simulink model "kaiguangai1108"  (R2016b)
settings: Solver=ode4  StartTime=0.0  StopTime=inf  FixedStep=0.002  RelTol=1e-3  EnableMultiTasking=on
libraries: slrtlib x5
(part 3 of 6)

== stateflow chart kaiguangai1108/Subsystem1/zidong/1# ==
  state zidong
    state chushihua
      entry:
      skhx=0;
      kghx=0;
      kgzhiling1=0;
      kgzhiling2=0;
      yjhx=0;
      gghx=0;
      ggzhiling1=0;
      ggzhiling2=0;
      skt=0;
      kgt=0;
      sdt=0;
      jst=0;
      ggt=0;
      yjt=0;
      skyichang=0;
      kgyichang=0;
      sdyichang=0;
      jsyichang=0;
      ggyichang=0;
      yjyichang=0;
    state on1
      entry:
      skhx=1;
    state songkaishijian
      entry:
      skt=skt+0.002;
    state start
      entry:
      yikaicishu = 0;
    state on10
      entry:
      skyichang=1;
    state songkaishijian1
      entry:
      skt=skt+0.002;
    state on8
      entry:
      skhx=0;
    state yanchishijian1
      entry:
      t=t+0.002;
    state tguiling
      entry: t=0;
    state on2
      entry:
      skhx=0;
      kghx=1;
      kgzhiling1=1;
      kgzhiling2=1;
    state kaigaishijian
      entry:
      kgt=kgt+0.002;
    state stop
      entry:
      skhx=0;
      kghx=0;
      kgzhiling1=0;
      kgzhiling2=0;
      yjhx=0;
      gghx=0;
      ggzhiling1=0;
      ggzhiling2=0;
      skt=0;
      kgt=0;
      sdt=0;
      jst=0;
      ggt=0;
      yjt=0;
    state songkaishijian2
      entry:
      kgt=kgt+0.002;
    state on9
      entry:
      kghx=0;
      kgzhiling1=0;
      kgzhiling2=0;
    state on11
      entry:
      kgyichang=1;
    state yanchishijian2
      entry:
      t2=t2+0.002;
    state t2guiling
      entry: t2=0;
    state on3
      entry:
      kghx=0;
      kgzhiling1=0;
      kgzhiling2=0;
      yjhx=1;
    state suodingshijian
      entry:
      sdt=sdt+0.002;
    state on7
      entry:
      yikaicishu = yikaicishu + 1;
    state songkaishijian3
      entry:
      sdt=sdt+0.002;
    state on13
      entry:
      yjhx=0;
    state on12
      entry:
      sdyichang=1;
    state yanchishijian3
      entry:
      t4=t4+0.002;
    state t4guiling
      entry: t4=0;
    state off
      entry:
      skhx=0;
      kghx=0;
      kgzhiling1=0;
      kgzhiling2=0;
      yjhx=0;
      gghx=0;
      ggzhiling1=0;
      ggzhiling2=0;
      skt=0;
    state on4
      entry:
      yjhx=0;
      skhx=1;
    state jiesuoshijian
      entry:
      jst=jst+0.002;
    state songkaishijian4
      entry:
      jst=jst+0.002;
    state on15
      entry:
      skhx=0;
    state on14
      entry:
      jsyichang=1;
    state yanchishijian4
      entry:
      t6=t6+0.002;
    state t6guiling
      entry: t6=0;
    state on5
      entry:
      skhx=0;
      gghx=1;
      ggzhiling1=1;
      ggzhiling2=1;
    state guangaishijian
      entry:
      ggt=ggt+0.002;
    state songkaishijian5
      entry:
      ggt=ggt+0.002;
    state on17
      entry:
      gghx=0;
      ggzhiling1=0;
      ggzhiling2=0;
    state on16
      entry:
      ggyichang=1;
    state yanchishijian5
      entry:
      t8=t8+0.002;
    state t8guiling
      entry: t8=0;
    state yanchishijian6
      entry:
      t10=t10+0.002;
    state on6
      entry:
      gghx=0;
      ggzhiling1=0;
      ggzhiling2=0;
      yjhx=1;
    state yajinshijian
      entry:
      yjt=yjt+0.002;
    state songkaishijian6
      entry:
      yjt=yjt+0.002;
    state on19
      entry:
      yjhx=0;
    state on18
      entry:
      ggyichang=1;
    state t10guiling
      entry: t10=0;
    (default) -> start
    chushihua -> on1 : [start==1&&ggdw1==1&&ggdw2==1&&yjdw==1&&sddw==1]
    songkaishijian1 -> songkaishijian1 [order 1] : [jsdw==0||skdw==0]
    on1 -> (junction 48)
    (junction 48) -> songkaishijian [order 1] : [jsdw==0||skdw==0]
    (junction 348) -> (junction 48) [order 1] : [skt<=2000]
    start -> chushihua : [start==1]
    (junction 48) -> tguiling [order 2] : [jsdw==1&&skdw==1]
    songkaishijian -> (junction 348)
    songkaishijian1 -> on8 [order 2] : [jsdw==1&&skdw==1]
    on10 -> songkaishijian1
    (junction 348) -> on10 [order 2] : [skt>2000]
    (junction 54) -> yanchishijian1 [order 1] : [t<t1]
    yanchishijian1 -> (junction 54) : after(1,tick)
    tguiling -> (junction 54)
    (junction 54) -> on2 [order 2] : [t>=t1]
    (junction 190) -> chushihua [order 1] : [yikaicishu<shedingcishu&&jieshu==0]
    songkaishijian2 -> songkaishijian2 [order 1] : [kgdw1==0||kgdw2==0||jsdw==0||skdw==0]
    on2 -> (junction 65)
    (junction 65) -> kaigaishijian [order 1] : [kgdw1==0||kgdw2==0||jsdw==0||skdw==0]
    (junction 361) -> (junction 65) [order 2] : [kgt<=12000]
    (junction 65) -> t2guiling [order 2] : [kgdw1==1&&kgdw2==1&&jsdw==1&&skdw==1]
    kaigaishijian -> (junction 361)
    (junction 76) -> yanchishijian2 [order 1] : [t2<t3]
    songkaishijian2 -> on9 [order 2] : [kgdw1==1&&kgdw2==1&&jsdw==1&&skdw==1]
    on11 -> songkaishijian2
    (junction 361) -> on11 [order 1] : [kgt>12000]
    (junction 190) -> stop [order 2] : [yikaicishu>=shedingcishu||jieshu==1]
    on7 -> (junction 190)
    yanchishijian2 -> (junction 76) : after(1,tick)
    t2guiling -> (junction 76)
    (junction 76) -> on3 [order 2] : [t2>=t3]
    songkaishijian3 -> songkaishijian3 [order 1] : [kgdw1==0||kgdw2==0||sddw==0||yjdw==0]
    on3 -> (junction 96)
    (junction 96) -> suodingshijian [order 1] : [kgdw1==0||kgdw2==0||sddw==0||yjdw==0]
    (junction 386) -> (junction 96) [order 2] : [sdt<=2000]
    (junction 96) -> t4guiling [order 2] : [kgdw1==1&&kgdw2==1&&sddw==1&&yjdw==1]
    off -> on7
    suodingshijian -> (junction 386)
    (junction 105) -> yanchishijian3 [order 1] : [t4<t5]
    songkaishijian3 -> on13 [order 2] : [kgdw1==1&&kgdw2==1&&jsdw==1&&skdw==1]
    on12 -> songkaishijian3
    (junction 386) -> on12 [order 1] : [sdt>2000]
    yanchishijian3 -> (junction 105) : after(1,tick)
    t4guiling -> (junction 105)
    (junction 105) -> on4 [order 2] : [t4>=t5]
    songkaishijian4 -> songkaishijian4 [order 1] : [kgdw1==0||kgdw2==0||jsdw==0||skdw==0]
    on4 -> (junction 115)
    (junction 115) -> jiesuoshijian [order 1] : [kgdw1==0||kgdw2==0||jsdw==0||skdw==0]
    (junction 390) -> (junction 115) [order 2] : [jst<=2000]
    (junction 115) -> t6guiling [order 2] : [kgdw1==1&&kgdw2==1&&jsdw==1&&skdw==1]
    (junction 339) -> off [order 2] : [t10>=t11]
    jiesuoshijian -> (junction 390)
    (junction 125) -> yanchishijian4 [order 1] : [t6<t7]
    songkaishijian4 -> on15 [order 2] : [kgdw1==1&&kgdw2==1&&jsdw==1&&skdw==1]
    on14 -> songkaishijian4
    (junction 390) -> on14 [order 1] : [jst>2000]
    yanchishijian4 -> (junction 125) : after(1,tick)
    t6guiling -> (junction 125)
    (junction 125) -> on5 [order 2] : [t6>=t7]
    songkaishijian5 -> songkaishijian5 [order 2] : [ggdw1==0||ggdw2==0||jsdw==0||skdw==0]
    on5 -> (junction 142)
    (junction 142) -> guangaishijian [order 1] : [ggdw1==0||ggdw2==0||jsdw==0||skdw==0]
    (junction 403) -> (junction 142) [order 2] : [ggt<=12000]
    (junction 142) -> t8guiling [order 2] : [ggdw1==1&&ggdw2==1&&jsdw==1&&skdw==1]
    guangaishijian -> (junction 403)
    (junction 154) -> yanchishijian5 [order 1] : [t8<t9]
    songkaishijian5 -> on17 [order 1] : [ggdw1==1&&ggdw2==1&&jsdw==1&&skdw==1]
    on16 -> songkaishijian5
    (junction 403) -> on16 [order 1] : [ggt>12000]
    yanchishijian5 -> (junction 154) : after(1,tick)
    t8guiling -> (junction 154)
    (junction 154) -> on6 [order 2] : [t8>=t9]
    yanchishijian6 -> (junction 339) : after(1,tick)
    (junction 339) -> yanchishijian6 [order 1] : [t10<t11]
    t10guiling -> (junction 339)
    on6 -> (junction 162)
    (junction 162) -> yajinshijian [order 1] : [sddw==0||yjdw==0]
    songkaishijian6 -> songkaishijian6 [order 2] : [sddw==0||yjdw==0]
    (junction 410) -> (junction 162) [order 2] : [yjt<=2000]
    (junction 162) -> t10guiling [order 2] : [sddw==1&&yjdw==1&&ggdw1==1&&ggdw2==1]
    yajinshijian -> (junction 410)
    songkaishijian6 -> on19 [order 1] : [sddw==1&&yjdw==1&&ggdw1==1&&ggdw2==1]
    on18 -> songkaishijian6
    (junction 410) -> on18 [order 1] : [yjt>2000]
  (default) -> zidong
  data: start input; kgdw1 input; kgdw2 input; skhx output; kghx output; kgzhiling1 output; kgzhiling2 output; yjhx output; gghx output; ggzhiling1 output; ggzhiling2 output; skt output; kgt output; sdt output; jst output; ggt output; yjt output; ggdw1 input; ggdw2 input; kghc input; gghc input; sddw input; jsdw input; yjdw input; skdw input; t1 input; t3 input; t5 input; t7 input; t9 input; t11 input; t local; t2 local; t4 local; t6 local; t8 local; shedingcishu input; yikaicishu output; skyichang output; kgyichang output; sdyichang output; jsyichang output; jieshu input; t10 local; ggyichang output; yjyichang output

== stateflow chart kaiguangai1108/Subsystem1/zidong/1#1 ==
  state zidong
    state chushihua
      entry:
      skhx=0;
      kghx=0;
      kgzhiling1=0;
      kgzhiling2=0;
      yjhx=0;
      gghx=0;
      ggzhiling1=0;
      ggzhiling2=0;
      skt=0;
      kgt=0;
      sdt=0;
      jst=0;
      ggt=0;
      yjt=0;
      skyichang=0;
      kgyichang=0;
      sdyichang=0;
      jsyichang=0;
      ggyichang=0;
      yjyichang=0;
    state on1
      entry:
      skhx=1;
    state songkaishijian
      entry:
      skt=skt+0.002;
    state start
      entry:
      yikaicishu = 0;
    state on10
      entry:
      skyichang=1;
    state songkaishijian1
      entry:
      skt=skt+0.002;
    state on8
      entry:
      skhx=0;
    state yanchishijian1
      entry:
      t=t+0.002;
    state tguiling
      entry: t=0;
    state on2
      entry:
      skhx=0;
      kghx=1;
      kgzhiling1=1;
      kgzhiling2=1;
    state kaigaishijian
      entry:
      kgt=kgt+0.002;
    state stop
      entry:
      skhx=0;
      kghx=0;
      kgzhiling1=0;
      kgzhiling2=0;
      yjhx=0;
      gghx=0;
      ggzhiling1=0;
      ggzhiling2=0;
      skt=0;
      kgt=0;
      sdt=0;
      jst=0;
      ggt=0;
      yjt=0;
    state songkaishijian2
      entry:
      kgt=kgt+0.002;
    state on9
      entry:
      kghx=0;
      kgzhiling1=0;
      kgzhiling2=0;
    state on11
      entry:
      kgyichang=1;
    state yanchishijian2
      entry:
      t2=t2+0.002;
    state t2guiling
      entry: t2=0;
    state on3
      entry:
      kghx=0;
      kgzhiling1=0;
      kgzhiling2=0;
      yjhx=1;
    state suodingshijian
      entry:
      sdt=sdt+0.002;
    state on7
      entry:
      yikaicishu = yikaicishu + 1;
    state songkaishijian3
      entry:
      sdt=sdt+0.002;
    state on13
      entry:
      yjhx=0;
    state on12
      entry:
      sdyichang=1;
    state yanchishijian3
      entry:
      t4=t4+0.002;
    state t4guiling
      entry: t4=0;
    state off
      entry:
      skhx=0;
      kghx=0;
      kgzhiling1=0;
      kgzhiling2=0;
      yjhx=0;
      gghx=0;
      ggzhiling1=0;
      ggzhiling2=0;
      skt=0;
      kgt=0;
      sdt=0;
      jst=0;
      ggt=0;
      yjt=0;
    state on4
      entry:
      yjhx=0;
      skhx=1;
    state jiesuoshijian
      entry:
      jst=jst+0.002;
    state songkaishijian4
      entry:
      jst=jst+0.002;
    state on15
      entry:
      skhx=0;
    state on14
      entry:
      jsyichang=1;
    state yanchishijian4
      entry:
      t6=t6+0.002;
    state t6guiling
      entry: t6=0;
    state on5
      entry:
      skhx=0;
      gghx=1;
      ggzhiling1=1;
      ggzhiling2=1;
    state guangaishijian
      entry:
      ggt=ggt+0.002;
    state songkaishijian5
      entry:
      ggt=ggt+0.002;
    state on17
      entry:
      gghx=0;
      ggzhiling1=0;
      ggzhiling2=0;
    state on16
      entry:
      ggyichang=1;
    state yanchishijian5
      entry:
      t8=t8+0.002;
    state t8guiling
      entry: t8=0;
    state yanchishijian6
      entry:
      t10=t10+0.002;
    state on6
      entry:
      gghx=0;
      ggzhiling1=0;
      ggzhiling2=0;
      yjhx=1;
    state yajinshijian
      entry:
      yjt=yjt+0.002;
    state songkaishijian6
      entry:
      yjt=yjt+0.002;
    state on19
      entry:
      yjhx=0;
    state on18
      entry:
      ggyichang=1;
    state t10guiling
      entry: t10=0;
    (default) -> start
    songkaishijian1 -> songkaishijian1 [order 1] : [jsdw==0||skdw==0]
    chushihua -> on1 : [start==1&&ggdw1==1&&ggdw2==1&&yjdw==1&&sddw==1]
    on1 -> (junction 48)
    (junction 48) -> songkaishijian [order 1] : [jsdw==0||skdw==0]
    start -> chushihua : [start==1]
    (junction 348) -> (junction 48) [order 1] : [skt<=2000]
    (junction 48) -> tguiling [order 2] : [jsdw==1&&skdw==1]
    songkaishijian -> (junction 348)
    songkaishijian1 -> on8 [order 2] : [jsdw==1&&skdw==1]
    on10 -> songkaishijian1
    (junction 348) -> on10 [order 2] : [skt>2000]
    (junction 54) -> yanchishijian1 [order 1] : [t<t1]
    yanchishijian1 -> (junction 54) : after(1,tick)
    tguiling -> (junction 54)
    (junction 54) -> on2 [order 2] : [t>=t1]
    (junction 190) -> chushihua [order 1] : [yikaicishu<shedingcishu&&jieshu==0]
    songkaishijian2 -> songkaishijian2 [order 1] : [kgdw1==0||kgdw2==0||jsdw==0||skdw==0]
    on2 -> (junction 65)
    (junction 65) -> kaigaishijian [order 1] : [kgdw1==0||kgdw2==0||jsdw==0||skdw==0]
    (junction 361) -> (junction 65) [order 2] : [kgt<=12000]
    (junction 65) -> t2guiling [order 2] : [kgdw1==1&&kgdw2==1&&jsdw==1&&skdw==1]
    kaigaishijian -> (junction 361)
    (junction 76) -> yanchishijian2 [order 1] : [t2<t3]
    songkaishijian2 -> on9 [order 2] : [kgdw1==1&&kgdw2==1&&jsdw==1&&skdw==1]
    on11 -> songkaishijian2
    (junction 361) -> on11 [order 1] : [kgt>12000]
    (junction 190) -> stop [order 2] : [yikaicishu>=shedingcishu||jieshu==1]
    on7 -> (junction 190)
    yanchishijian2 -> (junction 76) : after(1,tick)
    t2guiling -> (junction 76)
    (junction 76) -> on3 [order 2] : [t2>=t3]
    songkaishijian3 -> songkaishijian3 [order 1] : [kgdw1==0||kgdw2==0||sddw==0||yjdw==0]
    on3 -> (junction 96)
    (junction 96) -> suodingshijian [order 1] : [kgdw1==0||kgdw2==0||sddw==0||yjdw==0]
    (junction 386) -> (junction 96) [order 2] : [sdt<=2000]
    (junction 96) -> t4guiling [order 2] : [kgdw1==1&&kgdw2==1&&sddw==1&&yjdw==1]
    off -> on7
    suodingshijian -> (junction 386)
    (junction 105) -> yanchishijian3 [order 1] : [t4<t5]
    songkaishijian3 -> on13 [order 2] : [kgdw1==1&&kgdw2==1&&jsdw==1&&skdw==1]
    on12 -> songkaishijian3
    (junction 386) -> on12 [order 1] : [sdt>2000]
    yanchishijian3 -> (junction 105) : after(1,tick)
    t4guiling -> (junction 105)
    (junction 105) -> on4 [order 2] : [t4>=t5]
    songkaishijian4 -> songkaishijian4 [order 1] : [kgdw1==0||kgdw2==0||jsdw==0||skdw==0]
    on4 -> (junction 115)
    (junction 115) -> jiesuoshijian [order 1] : [kgdw1==0||kgdw2==0||jsdw==0||skdw==0]
    (junction 390) -> (junction 115) [order 2] : [jst<=2000]
    (junction 115) -> t6guiling [order 2] : [kgdw1==1&&kgdw2==1&&jsdw==1&&skdw==1]
    jiesuoshijian -> (junction 390)
    (junction 125) -> yanchishijian4 [order 1] : [t6<t7]
    songkaishijian4 -> on15 [order 2] : [kgdw1==1&&kgdw2==1&&jsdw==1&&skdw==1]
    on14 -> songkaishijian4
    (junction 390) -> on14 [order 1] : [jst>2000]
    yanchishijian4 -> (junction 125) : after(1,tick)
    t6guiling -> (junction 125)
    (junction 125) -> on5 [order 2] : [t6>=t7]
    (junction 339) -> off [order 2] : [t10>=t11]
    songkaishijian5 -> songkaishijian5 [order 2] : [ggdw1==0||ggdw2==0||jsdw==0||skdw==0]
    on5 -> (junction 142)
    (junction 142) -> guangaishijian [order 1] : [ggdw1==0||ggdw2==0||jsdw==0||skdw==0]
    (junction 403) -> (junction 142) [order 2] : [ggt<=12000]
    (junction 142) -> t8guiling [order 2] : [ggdw1==1&&ggdw2==1&&jsdw==1&&skdw==1]
    guangaishijian -> (junction 403)
    (junction 154) -> yanchishijian5 [order 1] : [t8<t9]
    songkaishijian5 -> on17 [order 1] : [ggdw1==1&&ggdw2==1&&jsdw==1&&skdw==1]
    on16 -> songkaishijian5
    (junction 403) -> on16 [order 1] : [ggt>12000]
    yanchishijian5 -> (junction 154) : after(1,tick)
    t8guiling -> (junction 154)
    (junction 154) -> on6 [order 2] : [t8>=t9]
    yanchishijian6 -> (junction 339) : after(1,tick)
    (junction 339) -> yanchishijian6 [order 1] : [t10<t11]
    t10guiling -> (junction 339)
    on6 -> (junction 162)
    (junction 162) -> yajinshijian [order 1] : [sddw==0||yjdw==0]
    songkaishijian6 -> songkaishijian6 [order 2] : [sddw==0||yjdw==0]
    (junction 410) -> (junction 162) [order 2] : [yjt<=2000]
    (junction 162) -> t10guiling [order 2] : [sddw==1&&yjdw==1&&ggdw1==1&&ggdw2==1]
    yajinshijian -> (junction 410)
    songkaishijian6 -> on19 [order 1] : [sddw==1&&yjdw==1&&ggdw1==1&&ggdw2==1]
    on18 -> songkaishijian6
    (junction 410) -> on18 [order 1] : [yjt>2000]
  (default) -> zidong
  data: start input; kgdw1 input; kgdw2 input; skhx output; kghx output; kgzhiling1 output; kgzhiling2 output; yjhx output; gghx output; ggzhiling1 output; ggzhiling2 output; skt output; kgt output; sdt output; jst output; ggt output; yjt output; ggdw1 input; ggdw2 input; kghc input; gghc input; sddw input; jsdw input; yjdw input; skdw input; t1 input; t3 input; t5 input; t7 input; t9 input; t11 input; t local; t2 local; t4 local; t6 local; t8 local; shedingcishu input; yikaicishu output; skyichang output; kgyichang output; sdyichang output; jsyichang output; jieshu input; t10 local; ggyichang output; yjyichang output

== stateflow chart kaiguangai1108/Subsystem1/zidong/1#2 ==
  state zidong
    state chushihua
      entry:
      skhx=0;
      kghx=0;
      kgzhiling1=0;
      kgzhiling2=0;
      yjhx=0;
      gghx=0;
      ggzhiling1=0;
      ggzhiling2=0;
      skt=0;
      kgt=0;
      sdt=0;
      jst=0;
      ggt=0;
      yjt=0;
      skyichang=0;
      kgyichang=0;
      sdyichang=0;
      jsyichang=0;
      ggyichang=0;
      yjyichang=0;
    state on1
      entry:
      skhx=1;
    state songkaishijian
      entry:
      skt=skt+0.002;
    state start
      entry:
      yikaicishu = 0;
    state on10
      entry:
      skyichang=1;
    state songkaishijian1
      entry:
      skt=skt+0.002;
    state on8
      entry:
      skhx=0;
    state yanchishijian1
      entry:
      t=t+0.002;
    state tguiling
      entry: t=0;
    state on2
      entry:
      skhx=0;
      kghx=1;
      kgzhiling1=1;
      kgzhiling2=1;
    state kaigaishijian
      entry:
      kgt=kgt+0.002;
    state stop
      entry:
      skhx=0;
      kghx=0;
      kgzhiling1=0;
      kgzhiling2=0;
      yjhx=0;
      gghx=0;
      ggzhiling1=0;
      ggzhiling2=0;
      skt=0;
      kgt=0;
      sdt=0;
      jst=0;
      ggt=0;
      yjt=0;
    state songkaishijian2
      entry:
      kgt=kgt+0.002;
    state on9
      entry:
      kghx=0;
      kgzhiling1=0;
      kgzhiling2=0;
    state on11
      entry:
      kgyichang=1;
    state yanchishijian2
      entry:
      t2=t2+0.002;
    state t2guiling
      entry: t2=0;
    state on3
      entry:
      kghx=0;
      kgzhiling1=0;
      kgzhiling2=0;
      yjhx=1;
    state suodingshijian
      entry:
      sdt=sdt+0.002;
    state on7
      entry:
      yikaicishu = yikaicishu + 1;
    state songkaishijian3
      entry:
      sdt=sdt+0.002;
    state on13
      entry:
      yjhx=0;
    state on12
      entry:
      sdyichang=1;
    state yanchishijian3
      entry:
      t4=t4+0.002;
    state t4guiling
      entry: t4=0;
    state off
      entry:
      skhx=0;
      kghx=0;
      kgzhiling1=0;
      kgzhiling2=0;
      yjhx=0;
      gghx=0;
      ggzhiling1=0;
      ggzhiling2=0;
      skt=0;
      kgt=0;
      sdt=0;
      jst=0;
      ggt=0;
      yjt=0;
    state on4
      entry:
      yjhx=0;
      skhx=1;
    state jiesuoshijian
      entry:
      jst=jst+0.002;
    state songkaishijian4
      entry:
      jst=jst+0.002;
    state on15
      entry:
      skhx=0;
    state on14
      entry:
      jsyichang=1;
    state yanchishijian4
      entry:
      t6=t6+0.002;
    state t6guiling
      entry: t6=0;
    state on5
      entry:
      skhx=0;
      gghx=1;
      ggzhiling1=1;
      ggzhiling2=1;
    state guangaishijian
      entry:
      ggt=ggt+0.002;
    state songkaishijian5
      entry:
      ggt=ggt+0.002;
    state on17
      entry:
      gghx=0;
      ggzhiling1=0;
      ggzhiling2=0;
    state on16
      entry:
      ggyichang=1;
    state yanchishijian5
      entry:
      t8=t8+0.002;
    state t8guiling
      entry: t8=0;
    state yanchishijian6
      entry:
      t10=t10+0.002;
    state on6
      entry:
      gghx=0;
      ggzhiling1=0;
      ggzhiling2=0;
      yjhx=1;
    state yajinshijian
      entry:
      yjt=yjt+0.002;
    state songkaishijian6
      entry:
      yjt=yjt+0.002;
    state on19
      entry:
      yjhx=0;
    state on18
      entry:
      ggyichang=1;
    state t10guiling
      entry: t10=0;
    (default) -> start
    songkaishijian1 -> songkaishijian1 [order 1] : [jsdw==0||skdw==0]
    chushihua -> on1 : [start==1&&ggdw1==1&&ggdw2==1&&yjdw==1&&sddw==1]
    on1 -> (junction 48)
    (junction 48) -> songkaishijian [order 1] : [jsdw==0||skdw==0]
    start -> chushihua : [start==1]
    (junction 348) -> (junction 48) [order 1] : [skt<=2000]
    (junction 48) -> tguiling [order 2] : [jsdw==1&&skdw==1]
    songkaishijian -> (junction 348)
    songkaishijian1 -> on8 [order 2] : [jsdw==1&&skdw==1]
    on10 -> songkaishijian1
    (junction 348) -> on10 [order 2] : [skt>2000]
    (junction 54) -> yanchishijian1 [order 1] : [t<t1]
    yanchishijian1 -> (junction 54) : after(1,tick)
    tguiling -> (junction 54)
    (junction 54) -> on2 [order 2] : [t>=t1]
    (junction 190) -> chushihua [order 1] : [yikaicishu<shedingcishu&&jieshu==0]
    songkaishijian2 -> songkaishijian2 [order 1] : [kgdw1==0||kgdw2==0||jsdw==0||skdw==0]
    on2 -> (junction 65)
    (junction 65) -> kaigaishijian [order 1] : [kgdw1==0||kgdw2==0||jsdw==0||skdw==0]
    (junction 361) -> (junction 65) [order 2] : [kgt<=12000]
    (junction 65) -> t2guiling [order 2] : [kgdw1==1&&kgdw2==1&&jsdw==1&&skdw==1]
    kaigaishijian -> (junction 361)
    (junction 76) -> yanchishijian2 [order 1] : [t2<t3]
    songkaishijian2 -> on9 [order 2] : [kgdw1==1&&kgdw2==1&&jsdw==1&&skdw==1]
    on11 -> songkaishijian2
    (junction 361) -> on11 [order 1] : [kgt>12000]
    (junction 190) -> stop [order 2] : [yikaicishu>=shedingcishu||jieshu==1]
    on7 -> (junction 190)
    yanchishijian2 -> (junction 76) : after(1,tick)
    t2guiling -> (junction 76)
    (junction 76) -> on3 [order 2] : [t2>=t3]
    songkaishijian3 -> songkaishijian3 [order 1] : [kgdw1==0||kgdw2==0||sddw==0||yjdw==0]
    on3 -> (junction 96)
    (junction 96) -> suodingshijian [order 1] : [kgdw1==0||kgdw2==0||sddw==0||yjdw==0]
    (junction 386) -> (junction 96) [order 2] : [sdt<=2000]
    (junction 96) -> t4guiling [order 2] : [kgdw1==1&&kgdw2==1&&sddw==1&&yjdw==1]
    off -> on7
    suodingshijian -> (junction 386)
    (junction 105) -> yanchishijian3 [order 1] : [t4<t5]
    songkaishijian3 -> on13 [order 2] : [kgdw1==1&&kgdw2==1&&jsdw==1&&skdw==1]
    on12 -> songkaishijian3
    (junction 386) -> on12 [order 1] : [sdt>2000]
    yanchishijian3 -> (junction 105) : after(1,tick)
    t4guiling -> (junction 105)
    (junction 105) -> on4 [order 2] : [t4>=t5]
    songkaishijian4 -> songkaishijian4 [order 1] : [kgdw1==0||kgdw2==0||jsdw==0||skdw==0]
    on4 -> (junction 115)
    (junction 115) -> jiesuoshijian [order 1] : [kgdw1==0||kgdw2==0||jsdw==0||skdw==0]
    (junction 390) -> (junction 115) [order 2] : [jst<=2000]
    (junction 115) -> t6guiling [order 2] : [kgdw1==1&&kgdw2==1&&jsdw==1&&skdw==1]
    jiesuoshijian -> (junction 390)
    (junction 125) -> yanchishijian4 [order 1] : [t6<t7]
    songkaishijian4 -> on15 [order 2] : [kgdw1==1&&kgdw2==1&&jsdw==1&&skdw==1]
    on14 -> songkaishijian4
    (junction 390) -> on14 [order 1] : [jst>2000]
    yanchishijian4 -> (junction 125) : after(1,tick)
    t6guiling -> (junction 125)
    (junction 125) -> on5 [order 2] : [t6>=t7]
    (junction 339) -> off [order 2] : [t10>=t11]
    songkaishijian5 -> songkaishijian5 [order 2] : [ggdw1==0||ggdw2==0||jsdw==0||skdw==0]
    on5 -> (junction 142)
    (junction 142) -> guangaishijian [order 1] : [ggdw1==0||ggdw2==0||jsdw==0||skdw==0]
    (junction 403) -> (junction 142) [order 2] : [ggt<=12000]
    (junction 142) -> t8guiling [order 2] : [ggdw1==1&&ggdw2==1&&jsdw==1&&skdw==1]
    guangaishijian -> (junction 403)
    (junction 154) -> yanchishijian5 [order 1] : [t8<t9]
    songkaishijian5 -> on17 [order 1] : [ggdw1==1&&ggdw2==1&&jsdw==1&&skdw==1]
    on16 -> songkaishijian5
    (junction 403) -> on16 [order 1] : [ggt>12000]
    yanchishijian5 -> (junction 154) : after(1,tick)
    t8guiling -> (junction 154)
    (junction 154) -> on6 [order 2] : [t8>=t9]
    yanchishijian6 -> (junction 339) : after(1,tick)
    (junction 339) -> yanchishijian6 [order 1] : [t10<t11]
    t10guiling -> (junction 339)
    on6 -> (junction 162)
    (junction 162) -> yajinshijian [order 1] : [sddw==0||yjdw==0]
    songkaishijian6 -> songkaishijian6 [order 2] : [sddw==0||yjdw==0]
    (junction 410) -> (junction 162) [order 2] : [yjt<=2000]
    (junction 162) -> t10guiling [order 2] : [sddw==1&&yjdw==1&&ggdw1==1&&ggdw2==1]
    yajinshijian -> (junction 410)
    songkaishijian6 -> on19 [order 1] : [sddw==1&&yjdw==1&&ggdw1==1&&ggdw2==1]
    on18 -> songkaishijian6
    (junction 410) -> on18 [order 1] : [yjt>2000]
  (default) -> zidong
  data: start input; kgdw1 input; kgdw2 input; skhx output; kghx output; kgzhiling1 output; kgzhiling2 output; yjhx output; gghx output; ggzhiling1 output; ggzhiling2 output; skt output; kgt output; sdt output; jst output; ggt output; yjt output; ggdw1 input; ggdw2 input; kghc input; gghc input; sddw input; jsdw input; yjdw input; skdw input; t1 input; t3 input; t5 input; t7 input; t9 input; t11 input; t local; t2 local; t4 local; t6 local; t8 local; shedingcishu input; yikaicishu output; skyichang output; kgyichang output; sdyichang output; jsyichang output; jieshu input; t10 local; ggyichang output; yjyichang output

== stateflow chart kaiguangai1108/Subsystem1/zidong/1#3 ==
  state zidong
    state chushihua
      entry:
      skhx=0;
      kghx=0;
      kgzhiling1=0;
      kgzhiling2=0;
      yjhx=0;
      gghx=0;
      ggzhiling1=0;
      ggzhiling2=0;
      skt=0;
      kgt=0;
      sdt=0;
      jst=0;
      ggt=0;
      yjt=0;
      skyichang=0;
      kgyichang=0;
      sdyichang=0;
      jsyichang=0;
      ggyichang=0;
      yjyichang=0;
    state on1
      entry:
      skhx=1;
    state songkaishijian
      entry:
      skt=skt+0.002;
    state start
      entry:
      yikaicishu = 0;
    state on10
      entry:
      skyichang=1;
    state songkaishijian1
      entry:
      skt=skt+0.002;
    state on8
      entry:
      skhx=0;
    state yanchishijian1
      entry:
      t=t+0.002;
    state tguiling
      entry: t=0;
    state on2
      entry:
      skhx=0;
      kghx=1;
      kgzhiling1=1;
      kgzhiling2=1;
    state kaigaishijian
      entry:
      kgt=kgt+0.002;
    state stop
      entry:
      skhx=0;
      kghx=0;
      kgzhiling1=0;
      kgzhiling2=0;
      yjhx=0;
      gghx=0;
      ggzhiling1=0;
      ggzhiling2=0;
      skt=0;
      kgt=0;
      sdt=0;
      jst=0;
      ggt=0;
      yjt=0;
    state songkaishijian2
      entry:
      kgt=kgt+0.002;
    state on9
      entry:
      kghx=0;
      kgzhiling1=0;
      kgzhiling2=0;
    state on11
      entry:
      kgyichang=1;
    state yanchishijian2
      entry:
      t2=t2+0.002;
    state t2guiling
      entry: t2=0;
    state on3
      entry:
      kghx=0;
      kgzhiling1=0;
      kgzhiling2=0;
      yjhx=1;
    state suodingshijian
      entry:
      sdt=sdt+0.002;
    state on7
      entry:
      yikaicishu = yikaicishu + 1;
    state songkaishijian3
      entry:
      sdt=sdt+0.002;
    state on13
      entry:
      yjhx=0;
    state on12
      entry:
      sdyichang=1;
    state yanchishijian3
      entry:
      t4=t4+0.002;
    state t4guiling
      entry: t4=0;
    state off
      entry:
      skhx=0;
      kghx=0;
      kgzhiling1=0;
      kgzhiling2=0;
      yjhx=0;
      gghx=0;
      ggzhiling1=0;
      ggzhiling2=0;
      skt=0;
      kgt=0;
      sdt=0;
      jst=0;
      ggt=0;
      yjt=0;
    state on4
      entry:
      yjhx=0;
      skhx=1;
    state jiesuoshijian
      entry:
      jst=jst+0.002;
    state songkaishijian4
      entry:
      jst=jst+0.002;
    state on15
      entry:
      skhx=0;
    state on14
      entry:
      jsyichang=1;
    state yanchishijian4
      entry:
      t6=t6+0.002;
    state t6guiling
      entry: t6=0;
    state on5
      entry:
      skhx=0;
      gghx=1;
      ggzhiling1=1;
      ggzhiling2=1;
    state guangaishijian
      entry:
      ggt=ggt+0.002;
    state songkaishijian5
      entry:
      ggt=ggt+0.002;
    state on17
      entry:
      gghx=0;
      ggzhiling1=0;
      ggzhiling2=0;
    state on16
      entry:
      ggyichang=1;
    state yanchishijian5
      entry:
      t8=t8+0.002;
    state t8guiling
      entry: t8=0;
    state yanchishijian6
      entry:
      t10=t10+0.002;
    state on6
      entry:
      gghx=0;
      ggzhiling1=0;
      ggzhiling2=0;
      yjhx=1;
    state yajinshijian
      entry:
      yjt=yjt+0.002;
    state songkaishijian6
      entry:
      yjt=yjt+0.002;
    state on19
      entry:
      yjhx=0;
    state on18
      entry:
      ggyichang=1;
    state t10guiling
      entry: t10=0;
    (default) -> start
    songkaishijian1 -> songkaishijian1 [order 1] : [jsdw==0||skdw==0]
    chushihua -> on1 : [start==1&&ggdw1==1&&ggdw2==1&&yjdw==1&&sddw==1]
    on1 -> (junction 48)
    (junction 48) -> songkaishijian [order 1] : [jsdw==0||skdw==0]
    start -> chushihua : [start==1]
    (junction 348) -> (junction 48) [order 1] : [skt<=2000]
    (junction 48) -> tguiling [order 2] : [jsdw==1&&skdw==1]
    songkaishijian -> (junction 348)
    songkaishijian1 -> on8 [order 2] : [jsdw==1&&skdw==1]
    on10 -> songkaishijian1
    (junction 348) -> on10 [order 2] : [skt>2000]
    (junction 54) -> yanchishijian1 [order 1] : [t<t1]
    yanchishijian1 -> (junction 54) : after(1,tick)
    tguiling -> (junction 54)
    (junction 54) -> on2 [order 2] : [t>=t1]
    (junction 190) -> chushihua [order 1] : [yikaicishu<shedingcishu&&jieshu==0]
    songkaishijian2 -> songkaishijian2 [order 1] : [kgdw1==0||kgdw2==0||jsdw==0||skdw==0]
    on2 -> (junction 65)
    (junction 65) -> kaigaishijian [order 1] : [kgdw1==0||kgdw2==0||jsdw==0||skdw==0]
    (junction 361) -> (junction 65) [order 2] : [kgt<=12000]
    (junction 65) -> t2guiling [order 2] : [kgdw1==1&&kgdw2==1&&jsdw==1&&skdw==1]
    kaigaishijian -> (junction 361)
    (junction 76) -> yanchishijian2 [order 1] : [t2<t3]
    songkaishijian2 -> on9 [order 2] : [kgdw1==1&&kgdw2==1&&jsdw==1&&skdw==1]
    on11 -> songkaishijian2
    (junction 361) -> on11 [order 1] : [kgt>12000]
    (junction 190) -> stop [order 2] : [yikaicishu>=shedingcishu||jieshu==1]
    on7 -> (junction 190)
    yanchishijian2 -> (junction 76) : after(1,tick)
    t2guiling -> (junction 76)
    (junction 76) -> on3 [order 2] : [t2>=t3]
    songkaishijian3 -> songkaishijian3 [order 1] : [kgdw1==0||kgdw2==0||sddw==0||yjdw==0]
    on3 -> (junction 96)
    (junction 96) -> suodingshijian [order 1] : [kgdw1==0||kgdw2==0||sddw==0||yjdw==0]
    (junction 386) -> (junction 96) [order 2] : [sdt<=2000]
    (junction 96) -> t4guiling [order 2] : [kgdw1==1&&kgdw2==1&&sddw==1&&yjdw==1]
    off -> on7
    suodingshijian -> (junction 386)
    (junction 105) -> yanchishijian3 [order 1] : [t4<t5]
    songkaishijian3 -> on13 [order 2] : [kgdw1==1&&kgdw2==1&&jsdw==1&&skdw==1]
    on12 -> songkaishijian3
    (junction 386) -> on12 [order 1] : [sdt>2000]
    yanchishijian3 -> (junction 105) : after(1,tick)
    t4guiling -> (junction 105)
    (junction 105) -> on4 [order 2] : [t4>=t5]
    songkaishijian4 -> songkaishijian4 [order 1] : [kgdw1==0||kgdw2==0||jsdw==0||skdw==0]
    on4 -> (junction 115)
    (junction 115) -> jiesuoshijian [order 1] : [kgdw1==0||kgdw2==0||jsdw==0||skdw==0]
    (junction 390) -> (junction 115) [order 2] : [jst<=2000]
    (junction 115) -> t6guiling [order 2] : [kgdw1==1&&kgdw2==1&&jsdw==1&&skdw==1]
    jiesuoshijian -> (junction 390)
    (junction 125) -> yanchishijian4 [order 1] : [t6<t7]
    songkaishijian4 -> on15 [order 2] : [kgdw1==1&&kgdw2==1&&jsdw==1&&skdw==1]
    on14 -> songkaishijian4
    (junction 390) -> on14 [order 1] : [jst>2000]
    yanchishijian4 -> (junction 125) : after(1,tick)
    t6guiling -> (junction 125)
    (junction 125) -> on5 [order 2] : [t6>=t7]
    (junction 339) -> off [order 2] : [t10>=t11]
    songkaishijian5 -> songkaishijian5 [order 2] : [ggdw1==0||ggdw2==0||jsdw==0||skdw==0]
    on5 -> (junction 142)
    (junction 142) -> guangaishijian [order 1] : [ggdw1==0||ggdw2==0||jsdw==0||skdw==0]
    (junction 403) -> (junction 142) [order 2] : [ggt<=12000]
    (junction 142) -> t8guiling [order 2] : [ggdw1==1&&ggdw2==1&&jsdw==1&&skdw==1]
    guangaishijian -> (junction 403)
    (junction 154) -> yanchishijian5 [order 1] : [t8<t9]
    songkaishijian5 -> on17 [order 1] : [ggdw1==1&&ggdw2==1&&jsdw==1&&skdw==1]
    on16 -> songkaishijian5
    (junction 403) -> on16 [order 1] : [ggt>12000]
    yanchishijian5 -> (junction 154) : after(1,tick)
    t8guiling -> (junction 154)
    (junction 154) -> on6 [order 2] : [t8>=t9]
    yanchishijian6 -> (junction 339) : after(1,tick)
    (junction 339) -> yanchishijian6 [order 1] : [t10<t11]
    t10guiling -> (junction 339)
    on6 -> (junction 162)
    (junction 162) -> yajinshijian [order 1] : [sddw==0||yjdw==0]
    songkaishijian6 -> songkaishijian6 [order 2] : [sddw==0||yjdw==0]
    (junction 410) -> (junction 162) [order 2] : [yjt<=2000]
    (junction 162) -> t10guiling [order 2] : [sddw==1&&yjdw==1&&ggdw1==1&&ggdw2==1]
    yajinshijian -> (junction 410)
    songkaishijian6 -> on19 [order 1] : [sddw==1&&yjdw==1&&ggdw1==1&&ggdw2==1]
    on18 -> songkaishijian6
    (junction 410) -> on18 [order 1] : [yjt>2000]
  (default) -> zidong
  data: start input; kgdw1 input; kgdw2 input; skhx output; kghx output; kgzhiling1 output; kgzhiling2 output; yjhx output; gghx output; ggzhiling1 output; ggzhiling2 output; skt output; kgt output; sdt output; jst output; ggt output; yjt output; ggdw1 input; ggdw2 input; kghc input; gghc input; sddw input; jsdw input; yjdw input; skdw input; t1 input; t3 input; t5 input; t7 input; t9 input; t11 input; t local; t2 local; t4 local; t6 local; t8 local; shedingcishu input; yikaicishu output; skyichang output; kgyichang output; sdyichang output; jsyichang output; jieshu input; t10 local; ggyichang output; yjyichang output

== stateflow chart kaiguangai1108/Subsystem1/zidong/1#4 ==
  state zidong
    state chushihua
      entry:
      skhx=0;
      kghx=0;
      kgzhiling1=0;
      kgzhiling2=0;
      yjhx=0;
      gghx=0;
      ggzhiling1=0;
      ggzhiling2=0;
      skt=0;
      kgt=0;
      sdt=0;
      jst=0;
      ggt=0;
      yjt=0;
      skyichang=0;
      kgyichang=0;
      sdyichang=0;
      jsyichang=0;
      ggyichang=0;
      yjyichang=0;
    state on1
      entry:
      skhx=1;
    state songkaishijian
      entry:
      skt=skt+0.002;
    state start
      entry:
      yikaicishu = 0;
    state on10
      entry:
      skyichang=1;
    state songkaishijian1
      entry:
      skt=skt+0.002;
    state on8
      entry:
      skhx=0;
    state yanchishijian1
      entry:
      t=t+0.002;
    state tguiling
      entry: t=0;
    state on2
      entry:
      skhx=0;
      kghx=1;
      kgzhiling1=1;
      kgzhiling2=1;
    state kaigaishijian
      entry:
      kgt=kgt+0.002;
    state stop
      entry:
      skhx=0;
      kghx=0;
      kgzhiling1=0;
      kgzhiling2=0;
      yjhx=0;
      gghx=0;
      ggzhiling1=0;
      ggzhiling2=0;
      skt=0;
      kgt=0;
      sdt=0;
      jst=0;
      ggt=0;
      yjt=0;
    state songkaishijian2
      entry:
      kgt=kgt+0.002;
    state on9
      entry:
      kghx=0;
      kgzhiling1=0;
      kgzhiling2=0;
    state on11
      entry:
      kgyichang=1;
    state yanchishijian2
      entry:
      t2=t2+0.002;
    state t2guiling
      entry: t2=0;
    state on3
      entry:
      kghx=0;
      kgzhiling1=0;
      kgzhiling2=0;
      yjhx=1;
    state suodingshijian
      entry:
      sdt=sdt+0.002;
    state on7
      entry:
      yikaicishu = yikaicishu + 1;
    state songkaishijian3
      entry:
      sdt=sdt+0.002;
    state on13
      entry:
      yjhx=0;
    state on12
      entry:
      sdyichang=1;
    state yanchishijian3
      entry:
      t4=t4+0.002;
    state t4guiling
      entry: t4=0;
    state off
      entry:
      skhx=0;
      kghx=0;
      kgzhiling1=0;
      kgzhiling2=0;
      yjhx=0;
      gghx=0;
      ggzhiling1=0;
      ggzhiling2=0;
      skt=0;
      kgt=0;
      sdt=0;
      jst=0;
      ggt=0;
      yjt=0;
    state on4
      entry:
      yjhx=0;
      skhx=1;
    state jiesuoshijian
      entry:
      jst=jst+0.002;
    state songkaishijian4
      entry:
      jst=jst+0.002;
    state on15
      entry:
      skhx=0;
    state on14
      entry:
      jsyichang=1;
    state yanchishijian4
      entry:
      t6=t6+0.002;
    state t6guiling
      entry: t6=0;
    state on5
      entry:
      skhx=0;
      gghx=1;
      ggzhiling1=1;
      ggzhiling2=1;
    state guangaishijian
      entry:
      ggt=ggt+0.002;
    state songkaishijian5
      entry:
      ggt=ggt+0.002;
    state on17
      entry:
      gghx=0;
      ggzhiling1=0;
      ggzhiling2=0;
    state on16
      entry:
      ggyichang=1;
    state yanchishijian5
      entry:
      t8=t8+0.002;
    state t8guiling
      entry: t8=0;
    state yanchishijian6
      entry:
      t10=t10+0.002;
    state on6
      entry:
      gghx=0;
      ggzhiling1=0;
      ggzhiling2=0;
      yjhx=1;
    state yajinshijian
      entry:
      yjt=yjt+0.002;
    state songkaishijian6
      entry:
      yjt=yjt+0.002;
    state on19
      entry:
      yjhx=0;
    state on18
      entry:
      ggyichang=1;
    state t10guiling
      entry: t10=0;
    (default) -> start
    songkaishijian1 -> songkaishijian1 [order 1] : [jsdw==0||skdw==0]
    chushihua -> on1 : [start==1&&ggdw1==1&&ggdw2==1&&yjdw==1&&sddw==1]
    on1 -> (junction 48)
    (junction 48) -> songkaishijian [order 1] : [jsdw==0||skdw==0]
    start -> chushihua : [start==1]
    (junction 348) -> (junction 48) [order 1] : [skt<=2000]
    (junction 48) -> tguiling [order 2] : [jsdw==1&&skdw==1]
    songkaishijian -> (junction 348)
    songkaishijian1 -> on8 [order 2] : [jsdw==1&&skdw==1]
    on10 -> songkaishijian1
    (junction 348) -> on10 [order 2] : [skt>2000]
    (junction 54) -> yanchishijian1 [order 1] : [t<t1]
    yanchishijian1 -> (junction 54) : after(1,tick)
    tguiling -> (junction 54)
    (junction 54) -> on2 [order 2] : [t>=t1]
    (junction 190) -> chushihua [order 1] : [yikaicishu<shedingcishu&&jieshu==0]
    songkaishijian2 -> songkaishijian2 [order 1] : [kgdw1==0||kgdw2==0||jsdw==0||skdw==0]
    on2 -> (junction 65)
    (junction 65) -> kaigaishijian [order 1] : [kgdw1==0||kgdw2==0||jsdw==0||skdw==0]
    (junction 361) -> (junction 65) [order 2] : [kgt<=12000]
    (junction 65) -> t2guiling [order 2] : [kgdw1==1&&kgdw2==1&&jsdw==1&&skdw==1]
    kaigaishijian -> (junction 361)
    (junction 76) -> yanchishijian2 [order 1] : [t2<t3]
    songkaishijian2 -> on9 [order 2] : [kgdw1==1&&kgdw2==1&&jsdw==1&&skdw==1]
    on11 -> songkaishijian2
    (junction 361) -> on11 [order 1] : [kgt>12000]
    (junction 190) -> stop [order 2] : [yikaicishu>=shedingcishu||jieshu==1]
    on7 -> (junction 190)
    yanchishijian2 -> (junction 76) : after(1,tick)
    t2guiling -> (junction 76)
    (junction 76) -> on3 [order 2] : [t2>=t3]
    songkaishijian3 -> songkaishijian3 [order 1] : [kgdw1==0||kgdw2==0||sddw==0||yjdw==0]
    on3 -> (junction 96)
    (junction 96) -> suodingshijian [order 1] : [kgdw1==0||kgdw2==0||sddw==0||yjdw==0]
    (junction 386) -> (junction 96) [order 2] : [sdt<=2000]
    (junction 96) -> t4guiling [order 2] : [kgdw1==1&&kgdw2==1&&sddw==1&&yjdw==1]
    off -> on7
    suodingshijian -> (junction 386)
    (junction 105) -> yanchishijian3 [order 1] : [t4<t5]
    songkaishijian3 -> on13 [order 2] : [kgdw1==1&&kgdw2==1&&jsdw==1&&skdw==1]
    on12 -> songkaishijian3
    (junction 386) -> on12 [order 1] : [sdt>2000]
    yanchishijian3 -> (junction 105) : after(1,tick)
    t4guiling -> (junction 105)
    (junction 105) -> on4 [order 2] : [t4>=t5]
    songkaishijian4 -> songkaishijian4 [order 1] : [kgdw1==0||kgdw2==0||jsdw==0||skdw==0]
    on4 -> (junction 115)
    (junction 115) -> jiesuoshijian [order 1] : [kgdw1==0||kgdw2==0||jsdw==0||skdw==0]
    (junction 390) -> (junction 115) [order 2] : [jst<=2000]
    (junction 115) -> t6guiling [order 2] : [kgdw1==1&&kgdw2==1&&jsdw==1&&skdw==1]
    jiesuoshijian -> (junction 390)
    (junction 125) -> yanchishijian4 [order 1] : [t6<t7]
    songkaishijian4 -> on15 [order 2] : [kgdw1==1&&kgdw2==1&&jsdw==1&&skdw==1]
    on14 -> songkaishijian4
    (junction 390) -> on14 [order 1] : [jst>2000]
    yanchishijian4 -> (junction 125) : after(1,tick)
    t6guiling -> (junction 125)
    (junction 125) -> on5 [order 2] : [t6>=t7]
    (junction 339) -> off [order 2] : [t10>=t11]
    songkaishijian5 -> songkaishijian5 [order 2] : [ggdw1==0||ggdw2==0||jsdw==0||skdw==0]
    on5 -> (junction 142)
    (junction 142) -> guangaishijian [order 1] : [ggdw1==0||ggdw2==0||jsdw==0||skdw==0]
    (junction 403) -> (junction 142) [order 2] : [ggt<=12000]
    (junction 142) -> t8guiling [order 2] : [ggdw1==1&&ggdw2==1&&jsdw==1&&skdw==1]
    guangaishijian -> (junction 403)
    (junction 154) -> yanchishijian5 [order 1] : [t8<t9]
    songkaishijian5 -> on17 [order 1] : [ggdw1==1&&ggdw2==1&&jsdw==1&&skdw==1]
    on16 -> songkaishijian5
    (junction 403) -> on16 [order 1] : [ggt>12000]
    yanchishijian5 -> (junction 154) : after(1,tick)
    t8guiling -> (junction 154)
    (junction 154) -> on6 [order 2] : [t8>=t9]
    yanchishijian6 -> (junction 339) : after(1,tick)
    (junction 339) -> yanchishijian6 [order 1] : [t10<t11]
    t10guiling -> (junction 339)
    on6 -> (junction 162)
    (junction 162) -> yajinshijian [order 1] : [sddw==0||yjdw==0]
    songkaishijian6 -> songkaishijian6 [order 2] : [sddw==0||yjdw==0]
    (junction 410) -> (junction 162) [order 2] : [yjt<=2000]
    (junction 162) -> t10guiling [order 2] : [sddw==1&&yjdw==1&&ggdw1==1&&ggdw2==1]
    yajinshijian -> (junction 410)
    songkaishijian6 -> on19 [order 1] : [sddw==1&&yjdw==1&&ggdw1==1&&ggdw2==1]
    on18 -> songkaishijian6
    (junction 410) -> on18 [order 1] : [yjt>2000]
  (default) -> zidong
  data: start input; kgdw1 input; kgdw2 input; skhx output; kghx output; kgzhiling1 output; kgzhiling2 output; yjhx output; gghx output; ggzhiling1 output; ggzhiling2 output; skt output; kgt output; sdt output; jst output; ggt output; yjt output; ggdw1 input; ggdw2 input; kghc input; gghc input; sddw input; jsdw input; yjdw input; skdw input; t1 input; t3 input; t5 input; t7 input; t9 input; t11 input; t local; t2 local; t4 local; t6 local; t8 local; shedingcishu input; yikaicishu output; skyichang output; kgyichang output; sdyichang output; jsyichang output; jieshu input; t10 local; ggyichang output; yjyichang output
